simulink model "HW01_model_2023_1112_PID"  (R2023a)
settings: Solver=ode45  StartTime=0.0  StopTime=150  RelTol=1e-3
libraries: slpidlib x1
settings Model: NumberOfSteps=10  PacingRate=10  Creator=YYlab_05  LastModifiedBy=YYlab_05

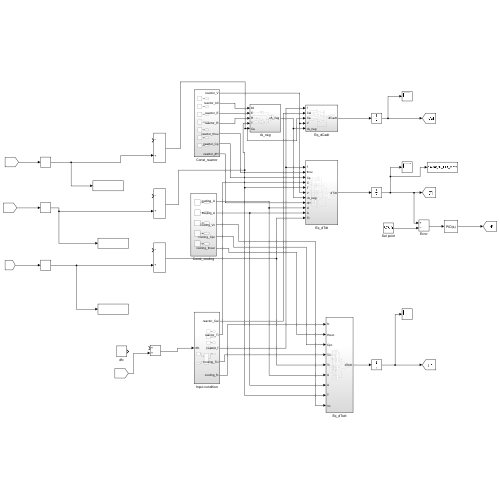
[thumbnail: Simulink's stored preview of the top-level diagram]
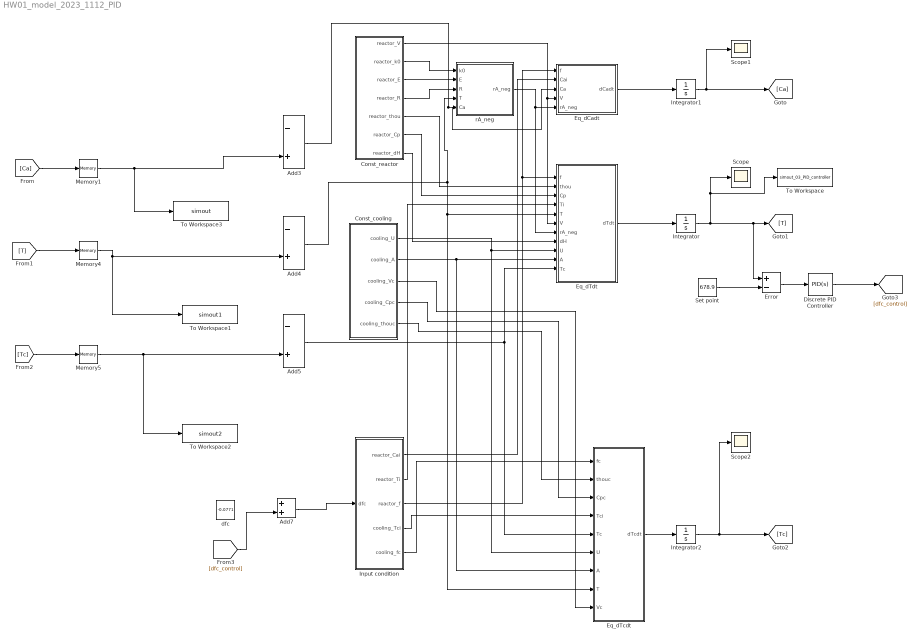
== system HW01_model_2023_1112_PID ==
  Add3 : Sum  Inputs=-+
  Add4 : Sum  Inputs=-+
  Add5 : Sum  Inputs=-+
  Add7 : Sum
  Const_cooling : Subsystem
  Const_reactor : Subsystem
  Discrete PID Controller : slpidlib/PID Controller  Controller=PID  Form=Parallel  TimeDomain=Continuous-time  UseExternalTs=off  SampleTime=-1  IntegratorMethod=Forward Euler  FilterMethod=Forward Euler  ControllerParametersSource=internal  P=-0.5566  I=2  UseKiTs=off  D=0.5  N=1  UseFilter=on  TunerSelectOption=Transfer Function Based (PID Tuner App)  InitialConditionSource=internal  InitialConditionForIntegrator=0  InitialConditionForFilter=0  DifferentiatorICPrevScaledInput=0  ExternalReset=none  TrackingMode=off  Kt=1  LimitOutput=off  SatLimitsSource=internal  UpperSaturationLimit=inf  LowerSaturationLimit=-inf  LinearizeAsGain=off  AntiWindupMode=none  Kb=1  LimitIntegrator=off  UpperIntegratorSaturationLimit=inf  LowerIntegratorSaturationLimit=-inf  POutMin=[]  POutMax=[]  IOutMin=[]  IOutMax=[]  DOutMin=[]  DOutMax=[]  NOutMin=[]  NOutMax=[]  SumOutMin=[]  SumOutMax=[]  SaturationOutMin=[]  SaturationOutMax=[]  PParamMin=[]  PParamMax=[]  IParamMin=[]  IParamMax=[]  DParamMin=[]  DParamMax=[]  NParamMin=[]  NParamMax=[]  KbParamMin=[]  KbParamMax=[]  KtParamMin=[]  KtParamMax=[]  KbOutMin=[]  KbOutMax=[]  KtOutMin=[]  KtOutMax=[]  IntegratorOutMin=[]  IntegratorOutMax=[]  FilterOutMin=[]  FilterOutMax=[]  SumI1OutMin=[]  SumI1OutMax=[]  SumI2OutMin=[]  SumI2OutMax=[]  SumI3OutMin=[]  SumI3OutMax=[]  SumI4OutMin=[]  SumI4OutMax=[]  SumDOutMin=[]  SumDOutMax=[]  DifferentiatorOutMin=[]  DifferentiatorOutMax=[]  FilterDiffOutCoefMin=[]  FilterDiffOutCoefMax=[]  ReciprocalOutMin=[]  ReciprocalOutMax=[]  SumDenOutMin=[]  SumDenOutMax=[]  SumNumOutMin=[]  SumNumOutMax=[]  DivideOutMin=[]  DivideOutMax=[]  UdiffTsProdOutMin=[]  UdiffTsProdOutMax=[]  NTsProdOutMin=[]  NTsProdOutMax=[]  UintegralTsProdOutMin=[]  UintegralTsProdOutMax=[]  UngainTsProdOutMin=[]  UngainTsProdOutMax=[]  ClampingZeroOutDataTypeStr=Inherit: Inherit via back propagation  ClampingZeroOutMin=[]  ClampingZeroOutMax=[]  FilterDenConstantOutDataTypeStr=Inherit: Inherit via back propagation  FilterDenConstantOutMin=[]  FilterDenConstantOutMax=[]  PCopyOutDataTypeStr=Inherit: Inherit via back propagation  PCopyOutMin=[]  PCopyOutMax=[]  NCopyOutDataTypeStr=Inherit: Inherit via back propagation  NCopyOutMin=[]  NCopyOutMax=[]  IntegratorContinuousStateAttributes=''  IntegratorStateMustResolveToSignalObject=off  IntegratorRTWStateStorageClass=Auto  FilterContinuousStateAttributes=''  FilterStateMustResolveToSignalObject=off  FilterRTWStateStorageClass=Auto  ParallelPVariant=InternalParameters  IdealPVariant=Disabled  IVariant=InternalParameters  DVariant=InternalParameters  IntegratorVariant=Continuous  SatVariant=Disabled  AWVariant=Passthrough  PCopyVariant=Disabled  TRVariant=Disabled  FdbkBlocksVariant=Forward  IdealPFdbkVariant=Disabled  SatFdbkVariant=Disabled  DerivativeFilterVariant=ContFilter  NVariant=InternalParameters  NCopyVariant=Disabled  FilterICVariant=InternalICsFilter  IntegratorICVariant=InternalICs  ExternalResetVariant=Disabled  TRSumVariant=Passthrough  SumFdbkVariant=Disabled  SumVariant=Sum_PID  TsampFilterVariant=InternalTs  TsampNgainVariant=Passthrough  TsampIntegralVariant=Disabled_SignalSpec  ExternalSaturationOutDataTypeStr=Inherit: Same as second input
      settings: LibrarySourceBlock=simulink/Discrete/Discrete PID Controller
  Eq_dCadt : Subsystem
  Eq_dTcdt : Subsystem
  Eq_dTdt : Subsystem
  Error : Sum  Inputs=+-
  Input condition : Subsystem
  Integrator : Integrator  InitialCondition=678.9
  Integrator1 : Integrator  InitialCondition=0.2068
  Integrator2 : Integrator  InitialCondition=602.7
  Memory1 : Memory  InitialCondition=0.2068
  Memory4 : Memory  InitialCondition=678.9
  Memory5 : Memory  InitialCondition=602.7
  Scope : Scope
  Scope1 : Scope
  Scope2 : Scope
  Set point : Constant  Value=678.9
  To Workspace : ToWorkspace  VariableName=simout_03_PID_controller  SaveFormat=Timeseries  SampleTime=-1
  To Workspace1 : ToWorkspace  VariableName=simout1  SaveFormat=Timeseries  SampleTime=-1
  To Workspace2 : ToWorkspace  VariableName=simout2  SaveFormat=Timeseries  SampleTime=-1
  To Workspace3 : ToWorkspace  VariableName=simout  SaveFormat=Timeseries  SampleTime=-1
  dfc : Constant  Value=-0.0771
  rA_neg : Subsystem
  wires:
  Const_reactor/2(reactor_k0) -> rA_neg/1(k0)
  Const_reactor/3(reactor_E) -> rA_neg/2(E)
  Const_reactor/4(reactor_R) -> rA_neg/3(R)
  Const_reactor/5(reactor_thou) -> Eq_dTdt/2(thou)
  Const_reactor/6(reactor_Cp) -> Eq_dTdt/3(Cp)
  Const_reactor/7(reactor_dH) -> Eq_dTdt/8(dH)
  rA_neg/1(rA_neg) -> Eq_dCadt/5(rA_neg), Eq_dTdt/7(rA_neg)
  Input condition/3(reactor_f) -> Eq_dTdt/1(f), Eq_dCadt/1(f)
  Input condition/1(reactor_Cai) -> Eq_dCadt/2(Cai)
  Const_reactor/1(reactor_V) -> Eq_dTdt/6(V), Eq_dCadt/4(V)
  Input condition/2(reactor_Ti) -> Eq_dTdt/4(Ti)
  Const_cooling/1(cooling_U) -> Eq_dTdt/9(U), Eq_dTcdt/6(U)
  Const_cooling/2(cooling_A) -> Eq_dTdt/10(A), Eq_dTcdt/7(A)
  Input condition/5(cooling_fc) -> Eq_dTcdt/1(fc)
  Const_cooling/5(cooling_thouc) -> Eq_dTcdt/2(thouc)
  Const_cooling/4(cooling_Cpc) -> Eq_dTcdt/3(Cpc)
  Input condition/4(cooling_Tci) -> Eq_dTcdt/4(Tci)
  Const_cooling/3(cooling_Vc) -> Eq_dTcdt/9(Vc)
  Eq_dTdt/1(dTdt) -> Integrator/1
  [T] -> Memory4/1
  [Tc] -> Memory5/1
  Add5/1 -> Eq_dTcdt/5(Tc), Eq_dTdt/11(Tc)
  Add4/1 -> rA_neg/4(T), Eq_dTcdt/8(T), Eq_dTdt/5(T)
  Add3/1 -> Eq_dCadt/3(Ca), rA_neg/5(Ca)
  Integrator/1 -> To Workspace/1, Scope/1, Error/1, [T]
  Integrator2/1 -> Scope2/1, [Tc]
  [Ca] -> Memory1/1
  Memory5/1 -> To Workspace2/1, Add5/2
  Eq_dTcdt/1(dTcdt) -> Integrator2/1
  Add7/1 -> Input condition/1(dfc)
  Memory4/1 -> To Workspace1/1, Add4/2
  Integrator1/1 -> Scope1/1, [Ca]
  Memory1/1 -> To Workspace3/1, Add3/2
  Eq_dCadt/1(dCadt) -> Integrator1/1
  Set point/1 -> Error/2
  Error/1 -> Discrete PID Controller/1
  Discrete PID Controller/1 -> [dfc_control]
  [dfc_control] -> Add7/2

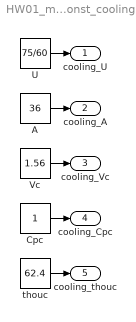
== system HW01_model_2023_1112_PID/Const_cooling ==
  A : Constant  Value=36
  Cpc : Constant
  U : Constant  Value=75/60
  Vc : Constant  Value=1.56
  thouc : Constant  Value=62.4
  cooling_U : Outport
  cooling_A : Outport  Port=2
  cooling_Vc : Outport  Port=3
  cooling_Cpc : Outport  Port=4
  cooling_thouc : Outport  Port=5
  wires:
  Vc/1 -> cooling_Vc/1
  Cpc/1 -> cooling_Cpc/1
  A/1 -> cooling_A/1
  U/1 -> cooling_U/1
  thouc/1 -> cooling_thouc/1

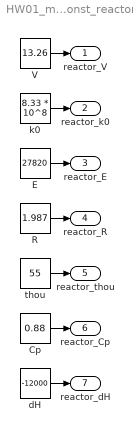
== system HW01_model_2023_1112_PID/Const_reactor ==
  Cp : Constant  Value=0.88
  E : Constant  Value=27820
  R : Constant  Value=1.987
  V : Constant  Value=13.26
  dH : Constant  Value=-12000  VectorParams1D=off
  k0 : Constant  Value=8.33 * 10^8
  thou : Constant  Value=55
  reactor_V : Outport
  reactor_k0 : Outport  Port=2
  reactor_E : Outport  Port=3
  reactor_R : Outport  Port=4
  reactor_thou : Outport  Port=5
  reactor_Cp : Outport  Port=6
  reactor_dH : Outport  Port=7
  wires:
  Cp/1 -> reactor_Cp/1
  V/1 -> reactor_V/1
  thou/1 -> reactor_thou/1
  k0/1 -> reactor_k0/1
  R/1 -> reactor_R/1
  E/1 -> reactor_E/1
  dH/1 -> reactor_dH/1

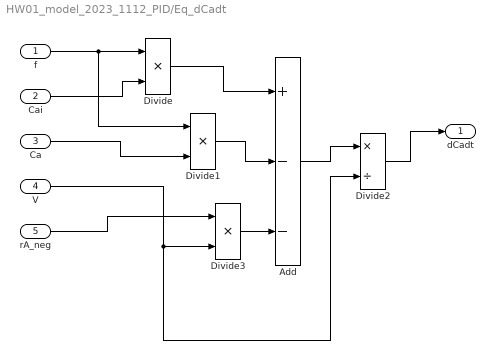
== system HW01_model_2023_1112_PID/Eq_dCadt ==
  f : Inport
  Cai : Inport  Port=2
  Ca : Inport  Port=3
  V : Inport  Port=4
  rA_neg : Inport  Port=5
  Add : Sum  Inputs=+--
  Divide : Product  Inputs=**
  Divide1 : Product  Inputs=**
  Divide2 : Product  Inputs=*/
  Divide3 : Product  Inputs=**
  dCadt : Outport
  wires:
  V/1 -> Divide2/2, Divide3/2
  rA_neg/1 -> Divide3/1
  Ca/1 -> Divide1/2
  f/1 -> Divide/1, Divide1/1
  Cai/1 -> Divide/2
  Divide/1 -> Add/1
  Divide1/1 -> Add/2
  Add/1 -> Divide2/1
  Divide2/1 -> dCadt/1
  Divide3/1 -> Add/3

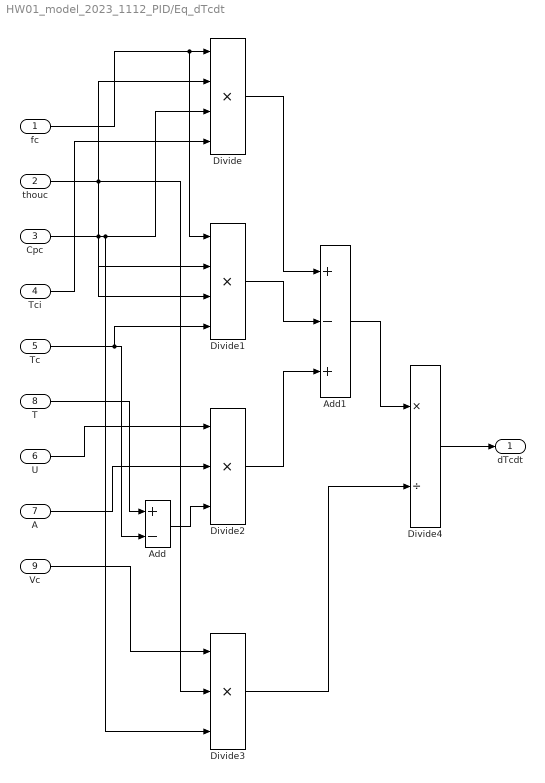
== system HW01_model_2023_1112_PID/Eq_dTcdt ==
  fc : Inport
  thouc : Inport  Port=2
  Cpc : Inport  Port=3
  Tci : Inport  Port=4
  Tc : Inport  Port=5
  U : Inport  Port=6
  A : Inport  Port=7
  T : Inport  Port=8
  Vc : Inport  Port=9
  Add : Sum  Inputs=+-
  Add1 : Sum  Inputs=+-+
  Divide : Product  Inputs=****
  Divide1 : Product  Inputs=****
  Divide2 : Product  Inputs=***
  Divide3 : Product  Inputs=***
  Divide4 : Product  Inputs=*/
  dTcdt : Outport
  wires:
  fc/1 -> Divide/1, Divide1/1
  thouc/1 -> Divide1/2, Divide/2, Divide3/2
  Cpc/1 -> Divide/3, Divide3/3, Divide1/3
  Tci/1 -> Divide/4
  Tc/1 -> Add/2, Divide1/4
  U/1 -> Divide2/1
  A/1 -> Divide2/2
  Add/1 -> Divide2/3
  T/1 -> Add/1
  Vc/1 -> Divide3/1
  Divide/1 -> Add1/1
  Divide1/1 -> Add1/2
  Divide2/1 -> Add1/3
  Add1/1 -> Divide4/1
  Divide3/1 -> Divide4/2
  Divide4/1 -> dTcdt/1

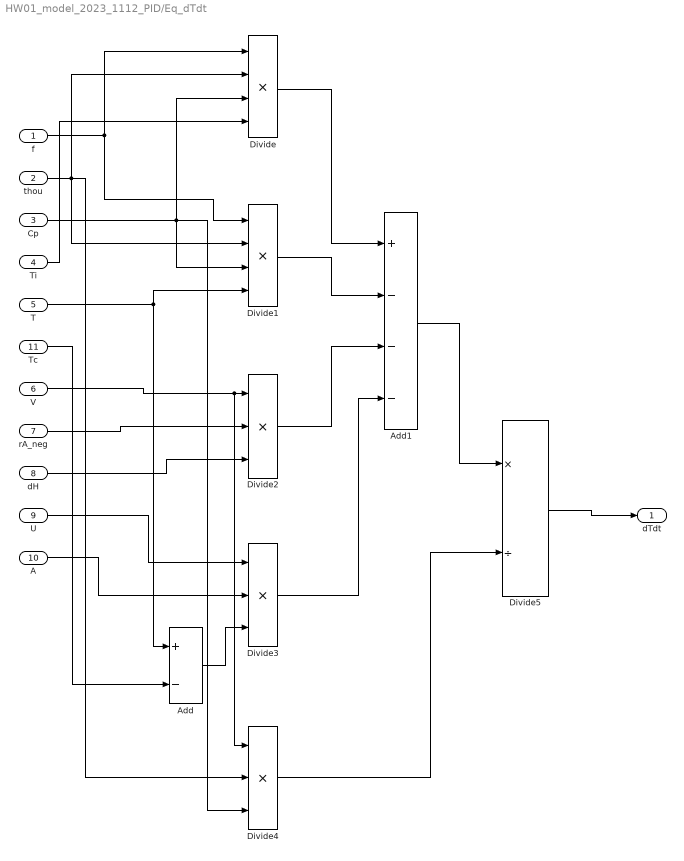
== system HW01_model_2023_1112_PID/Eq_dTdt ==
  f : Inport
  thou : Inport  Port=2
  Cp : Inport  Port=3
  Ti : Inport  Port=4
  T : Inport  Port=5
  V : Inport  Port=6
  rA_neg : Inport  Port=7
  dH : Inport  Port=8
  U : Inport  Port=9
  A : Inport  Port=10
  Tc : Inport  Port=11
  Add : Sum  Inputs=+-
  Add1 : Sum  Inputs=+---
  Divide : Product  Inputs=****
  Divide1 : Product  Inputs=****
  Divide2 : Product  Inputs=***
  Divide3 : Product  Inputs=***
  Divide4 : Product  Inputs=***
  Divide5 : Product  Inputs=*/
  dTdt : Outport
  wires:
  f/1 -> Divide1/1, Divide/1
  thou/1 -> Divide1/2, Divide/2, Divide4/2
  Cp/1 -> Divide1/3, Divide/3, Divide4/3
  Ti/1 -> Divide/4
  T/1 -> Add/1, Divide1/4
  V/1 -> Divide4/1, Divide2/1
  rA_neg/1 -> Divide2/2
  dH/1 -> Divide2/3
  U/1 -> Divide3/1
  A/1 -> Divide3/2
  Tc/1 -> Add/2
  Add/1 -> Divide3/3
  Divide/1 -> Add1/1
  Divide1/1 -> Add1/2
  Divide2/1 -> Add1/3
  Divide3/1 -> Add1/4
  Add1/1 -> Divide5/1
  Divide4/1 -> Divide5/2
  Divide5/1 -> dTdt/1

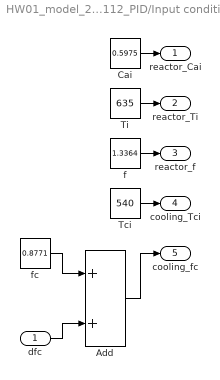
== system HW01_model_2023_1112_PID/Input condition ==
  dfc : Inport
  Add : Sum
  Cai : Constant  Value=0.5975
  Tci : Constant  Value=540
  Ti : Constant  Value=635
  f : Constant  Value=1.3364
  fc : Constant  Value=0.8771  VectorParams1D=off
  reactor_Cai : Outport
  reactor_Ti : Outport  Port=2
  reactor_f : Outport  Port=3
  cooling_Tci : Outport  Port=4
  cooling_fc : Outport  Port=5
  wires:
  Ti/1 -> reactor_Ti/1
  Cai/1 -> reactor_Cai/1
  f/1 -> reactor_f/1
  Tci/1 -> cooling_Tci/1
  fc/1 -> Add/1
  dfc/1 -> Add/2
  Add/1 -> cooling_fc/1

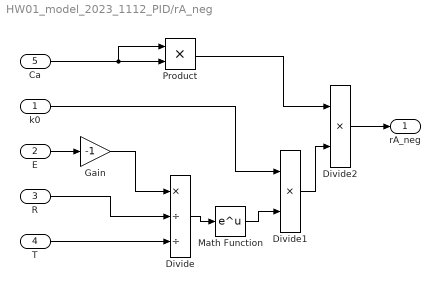
== system HW01_model_2023_1112_PID/rA_neg ==
  k0 : Inport
  E : Inport  Port=2
  R : Inport  Port=3
  T : Inport  Port=4
  Ca : Inport  Port=5
  Divide : Product  Inputs=*//
  Divide1 : Product  Inputs=**
  Divide2 : Product  Inputs=**
  Gain : Gain  Gain=-1
  Math Function : Math
  Product : Product
  rA_neg : Outport
  wires:
  Divide/1 -> Math Function/1
  E/1 -> Gain/1
  Gain/1 -> Divide/1
  R/1 -> Divide/2
  T/1 -> Divide/3
  Math Function/1 -> Divide1/2
  k0/1 -> Divide1/1
  Divide2/1 -> rA_neg/1
  Ca/1 -> Product/2, Product/1
  Divide1/1 -> Divide2/2
  Product/1 -> Divide2/1
